simulink model "heconlacnguoc"  (R2019a)
settings: Solver=ode5  StartTime=0.0  StopTime=10  FixedStep=0.01  RelTol=1e-3  EnableMultiTasking=on
undefined symbols (not defined in the file): sigbuilder_block
libraries: fuzblock x1
settings Model: Creator=ADMIN  LastModifiedBy=forev
settings DataIOCC: LimitDataPoints=on  SaveFormat=Array  SignalLoggingSaveFormat=ModelDataLogs  ReturnWorkspaceOutputs=off
settings OptimizationCC: ExpressionDepthLimit=2147483647  LifeSpan=inf
settings DebuggingCC: AlgebraicLoopMsg=none  UnderspecifiedInitializationDetection=Classic  MergeDetectMultiDrivingBlocksExec=none  SolverPrmCheckMsg=warning  FcnCallInpInsideContextMsg=warning  StateNameClashWarn=warning  SFUnexpectedBacktrackingDiag=warning  SFNoUnconditionalDefaultTransitionDiag=warning  SFExecutionAtInitializationDiag=none  ArithmeticOperatorsInVariantConditions=warning
settings HardwareCC: ProdBitPerPointer=32  ProdBitPerSizeT=32  ProdBitPerPtrDiffT=32  ProdLargestAtomicFloat=None  ProdIntDivRoundTo=Undefined  ProdEndianess=Unspecified  ProdWordSize=32  ProdHWDeviceType=32-bit Generic
settings ModelReferenceCC: PropagateSignalLabelsOutOfModel=off
settings SFSimCC: SimUseLocalCustomCode=off
settings RTWCC: RTWUseLocalCustomCode=off
settings CodeAppCC: StateflowObjectComments=on
settings GRTTargetCC: TargetLangStandard=C89/C90 (ANSI)  GeneratePreprocessorConditionals=Disable all  CombineOutputUpdateFcns=off  GRTInterface=on
settings ConfigComp: CovMetricSettings=dw  CovHtmlReporting=on  CovSaveCumulativeToWorkspaceVar=on  CovSaveSingleToWorkspaceVar=on  CovExternalEMLEnable=off

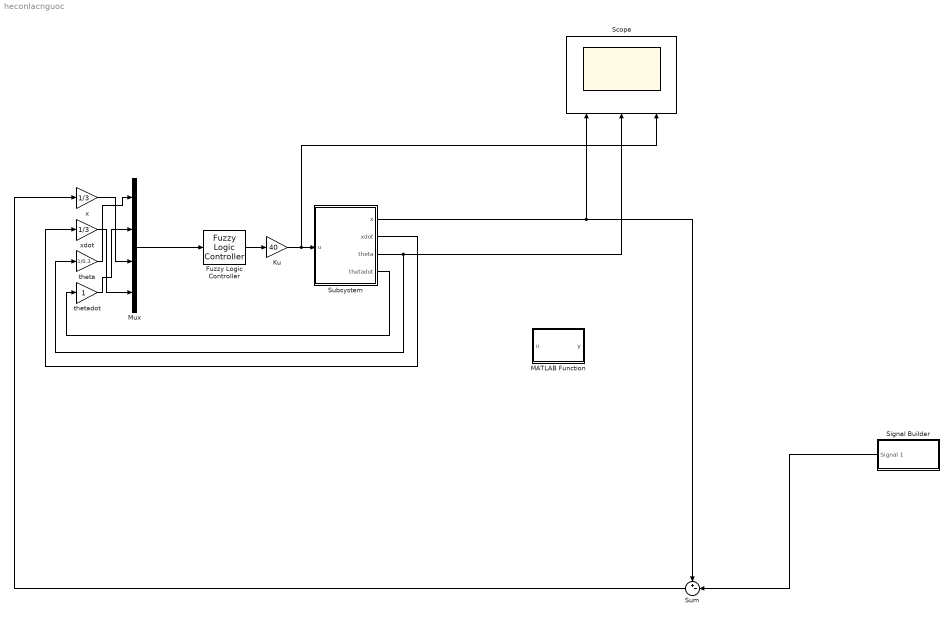
== system heconlacnguoc ==
  Fuzzy Logic Controller : fuzblock/Fuzzy Logic  Controller  FIS='fuzzy_rule.fis'  OutputSampleNumber=101  DataType=double  FuzzifiedInputs=off  RuleFiringStrengths=off  RuleOutputs=off  AggregatedOutputs=off  SimulateUsing=Interpreted execution  OutOfRangeInputValueMessage=warning  NoRuleFiredMessage=warning  EmptyOutputFuzzySetMessage=warning
  Ku : Gain  Gain=40
  MATLAB Function : MATLAB Function  TreatAsAtomicUnit=on
  Mux : Mux
  Scope : Scope  NumInputPorts=3
  Signal Builder : Subsystem  Tag=STV Subsys  LoadFcn=sigbuilder_block('load');  StartFcn=sigbuilder_block('start');  StopFcn=sigbuilder_block('stop');  ClipboardFcn=sigbuilder_block('clipboard');  mask(Sigbuilder block){tuvar=[0:10]}
      mask help: Simulink:masks:SigbuilderBlock_MD
      mask init:
      | if ~strcmp(get_param(bdroot(gcbh),'SimulationStatus'),'stopped') tuvar = sigbuilder_block('maskInit'); end
      settings: CopyFcn=sigbuilder_block('copy');  DeleteFcn=sigbuilder_block('delete');  ModelCloseFcn=sigbuilder_block('modelClose');  PreSaveFcn=sigbuilder_block('preSave');  PauseFcn=sigbuilder_block('pause');  ContinueFcn=sigbuilder_block('continue');  NameChangeFcn=sigbuilder_block('namechange');  OpenFcn=sigbuilder_block('open',[5.4 30 1141.2 522.6 ]);  CloseFcn=sigbuilder_block('close');
      mask Display: plot(0, 0, 100, 100,[2, 2, 32, 32, 2], [68, 8, 8, 68, 68],[32, 2], [38, 38], [32, 19, 2],[53, 60, 44], [32, 17, 17, 2],[16, 16, 31, 31]);txt = getActiveGroup(gcbh);text(2, 100, txt,'verticalAlignment', 'top');
  Subsystem : Subsystem  mask{M=1, k=0.1, l=0.5, g=9.81, x0=0, x_dot0=0, theta0=pi/6, theta_dot0=0}
      mask prompts: M "trọng lượng xe"; k "trong lượng con lắc"; l "chiều dài con lắc"; g "gia tốc trọng trường"; x0 "vị trí ban đầu"; x_dot0 "vận tốc ban đầu"; theta0 "góc lệch ban đầu"; theta_dot0 "vận tốc góc ban đầu"
  Sum : Sum  Inputs=+-|
  theta : Gain  Gain=1/0.3
  thetadot : Gain
  x : Gain  Gain=1/3
  xdot : Gain  Gain=1/3
  wires:
  Fuzzy Logic Controller/1 -> Ku/1
  Ku/1 -> Scope/3, Subsystem/1(u)
  Subsystem/2(xdot) -> xdot/1
  Subsystem/3(theta) -> theta/1, Scope/2
  Subsystem/4(thetadot) -> thetadot/1
  Mux/1 -> Fuzzy Logic Controller/1
  Subsystem/1(x) -> Sum/1, Scope/1
  Sum/1 -> x/1
  Signal Builder/1(Signal 1) -> Sum/2
  x/1 -> Mux/3
  xdot/1 -> Mux/4
  theta/1 -> Mux/1
  thetadot/1 -> Mux/2

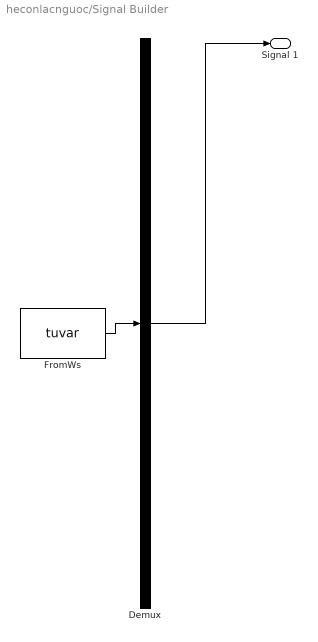
== system heconlacnguoc/Signal Builder ==
  Demux : Demux  Tag=STV Demux  Outputs=1
  FromWs : FromWorkspace  Tag=STV FromWs  VariableName=tuvar  SampleTime=0
      SigBuilderData=|
      | common.afterFinalStr = 'Extrapolate'
      | common.sampleTime = 0
      | dataSet.timeRange = [0 20]
      | dataSet.name = 'Group 1'
      | sbobj.Groups.Name = 'Group 1'
      | sbobj.Groups.Signals.Name = 'Signal 1'
      | sbobj.Groups.Signals.XData = [0 9.98 9.98 20]
      | sbobj.Groups.Signals.YData = [0.5 0.5 0 0]
      | sbobj.Groups.TimeRange = [0 20]
  Signal 1 : Outport  Tag=STV Outport
  wires:
  Demux/1 -> Signal 1/1
  FromWs/1 -> Demux/1

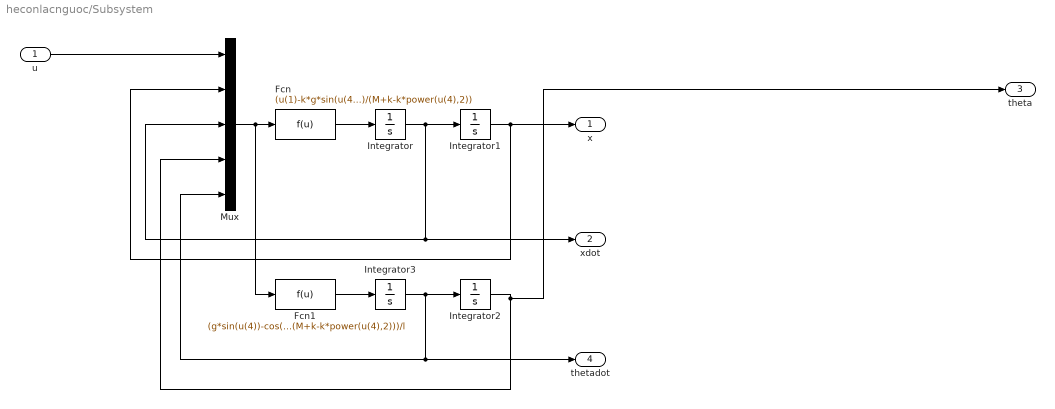
== system heconlacnguoc/Subsystem ==
  u : Inport
  Fcn : Fcn  Expr=(u(1)-k*g*sin(u(4))*cos(u(4))+k*l*sin(u(4))*power(u(5),2))/(M+k-k*power(u(4),2))
  Fcn1 : Fcn  Expr=(g*sin(u(4))-cos(u(4))*(u(1)-k*g*sin(u(4))*cos(u(4))+k*l*sin(u(4))*power(u(5),2))/(M+k-k*power(u(4),2)))/l
  Integrator : Integrator  InitialCondition=x_dot0
  Integrator1 : Integrator  InitialCondition=x0
  Integrator2 : Integrator  InitialCondition=theta0
  Integrator3 : Integrator  InitialCondition=theta_dot0
  Mux : Mux  Inputs=5
  x : Outport
  xdot : Outport  Port=2
  theta : Outport  Port=3
  thetadot : Outport  Port=4
  wires:
  Fcn1/1 -> Integrator3/1
  Integrator2/1 -> theta/1, Mux/4
  Integrator/1 -> Integrator1/1, xdot/1, Mux/3
  Mux/1 -> Fcn/1, Fcn1/1
  Integrator3/1 -> Integrator2/1, thetadot/1, Mux/5
  u/1 -> Mux/1
  Integrator1/1 -> x/1, Mux/2
  Fcn/1 -> Integrator/1

== matlab function heconlacnguoc/MATLAB Function ==
  data: u input; y output
function y = fcn(u)
t = mod(u,2*pi);
if(t>pi)
    y=t-2*pi;
else
    y=t;
end
end
